simulink model "pv_simulink"  (R2025b)
settings: Solver=ode45  StartTime=0.0  StopTime=604900  RelTol=1e-3
InitFcn:
  | modellDatei   = get_param('pv_simulink', 'FileName');
  | projektWurzel = fileparts(fileparts(modellDatei));
  | addpath(projektWurzel);
  | 
  | p = init_parameters();
undefined symbols (not defined in the file): Tm_start
settings Model: Creator=T450s  LastModifiedBy=T450s

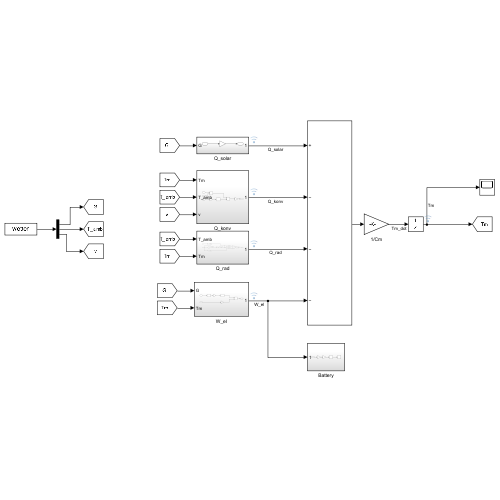
[thumbnail: Simulink's stored preview of the top-level diagram]
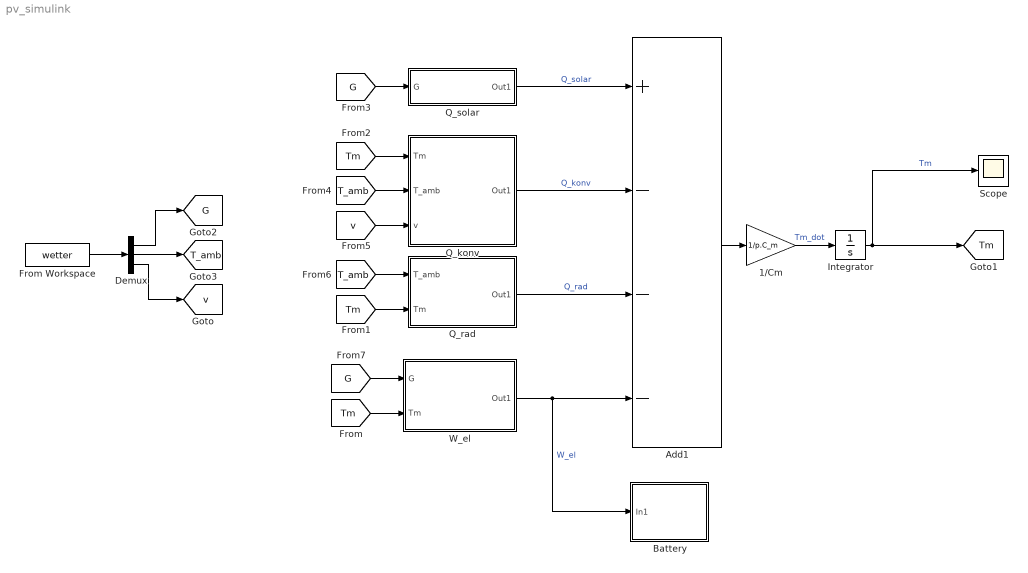
== system pv_simulink ==
  1/Cm : Gain  Gain=1/p.C_m
  Add1 : Sum  Inputs=+---
  Battery : Subsystem
  Demux : Demux  Outputs=3
  From Workspace : FromWorkspace  VariableName=wetter
  Integrator : Integrator  InitialCondition=Tm_start
  Q_konv : Subsystem
  Q_rad : Subsystem
  Q_solar : Subsystem
  Scope : Scope
      settings: ActiveDisplayYMinimum=-1  ActiveDisplayYMaximum=1
  W_el : Subsystem
  tag scope: G=global, T_amb=global, Tm=global, v=global
  wires:
  1/Cm/1 -> Integrator/1  "Tm_dot"
  Add1/1 -> 1/Cm/1
  Q_rad/1(Out1) -> Add1/3  "Q_rad"
  W_el/1(Out1) -> Battery/1(In1), Add1/4  "W_el"
  Q_konv/1(Out1) -> Add1/2  "Q_konv"
  Q_solar/1(Out1) -> Add1/1  "Q_solar"
  Integrator/1 -> Scope/1, [Tm]  "Tm"
  [Tm] -> W_el/2(Tm)
  [Tm] -> Q_rad/2(Tm)
  [Tm] -> Q_konv/1(Tm)
  [G] -> Q_solar/1(G)
  [T_amb] -> Q_konv/2(T_amb)
  [v] -> Q_konv/3(v)
  [T_amb] -> Q_rad/1(T_amb)
  [G] -> W_el/1(G)
  From Workspace/1 -> Demux/1
  Demux/1 -> [G]
  Demux/2 -> [T_amb]
  Demux/3 -> [v]

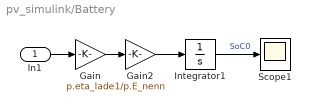
== system pv_simulink/Battery ==
  In1 : Inport
  Gain : Gain  Gain=p.eta_lade
  Gain2 : Gain  Gain=1/p.E_nenn
  Integrator1 : Integrator  InitialCondition=p.SoC0  LimitOutput=on  UpperSaturationLimit=1  LowerSaturationLimit=0
  Scope1 : Scope
      settings: ActiveDisplayYMinimum=0.10000000000000003  ActiveDisplayYMaximum=1.1
  wires:
  Gain2/1 -> Integrator1/1
  Gain/1 -> Gain2/1
  Integrator1/1 -> Scope1/1  "SoC0"
  In1/1 -> Gain/1

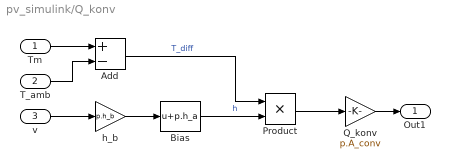
== system pv_simulink/Q_konv ==
  Tm : Inport
  T_amb : Inport  Port=2
  v : Inport  Port=3
  Add : Sum  Inputs=+-
  Bias : Bias  Bias=p.h_a  SaturateOnIntegerOverflow=off
  Product : Product
  Q_konv : Gain  Gain=p.A_conv
  h_b : Gain  Gain=p.h_b
  Out1 : Outport
  wires:
  T_amb/1 -> Add/2
  Add/1 -> Product/1  "T_diff"
  h_b/1 -> Bias/1
  Bias/1 -> Product/2  "h"
  Product/1 -> Q_konv/1
  Q_konv/1 -> Out1/1
  Tm/1 -> Add/1
  v/1 -> h_b/1

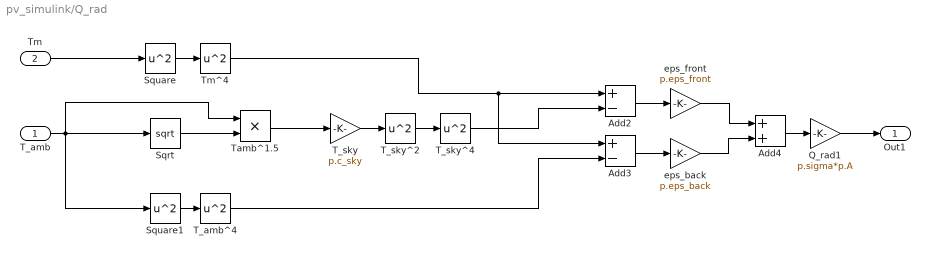
== system pv_simulink/Q_rad ==
  T_amb : Inport
  Tm : Inport  Port=2
  Add2 : Sum  Inputs=+-
  Add3 : Sum  Inputs=+-
  Add4 : Sum
  Q_rad1 : Gain  Gain=p.sigma*p.A
  Sqrt : Sqrt
  Square : Math  Operator=square
  Square1 : Math  Operator=square
  T_amb^4 : Math  Operator=square
  T_sky : Gain  Gain=p.c_sky
  T_sky^2 : Math  Operator=square
  T_sky^4 : Math  Operator=square
  Tamb^1.5 : Product
  Tm^4 : Math  Operator=square
  eps_back : Gain  Gain=p.eps_back
  eps_front : Gain  Gain=p.eps_front
  Out1 : Outport
  wires:
  eps_back/1 -> Add4/2
  T_amb^4/1 -> Add3/2
  Add3/1 -> eps_back/1
  Square1/1 -> T_amb^4/1
  Square/1 -> Tm^4/1
  Tamb^1.5/1 -> T_sky/1
  eps_front/1 -> Add4/1
  T_sky^4/1 -> Add2/2
  T_sky/1 -> T_sky^2/1
  Tm^4/1 -> Add3/1, Add2/1
  Add4/1 -> Q_rad1/1
  Sqrt/1 -> Tamb^1.5/2
  T_sky^2/1 -> T_sky^4/1
  Add2/1 -> eps_front/1
  T_amb/1 -> Tamb^1.5/1, Square1/1, Sqrt/1
  Q_rad1/1 -> Out1/1
  Tm/1 -> Square/1

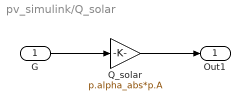
== system pv_simulink/Q_solar ==
  G : Inport
  Q_solar : Gain  Gain=p.alpha_abs*p.A
  Out1 : Outport
  wires:
  G/1 -> Q_solar/1
  Q_solar/1 -> Out1/1

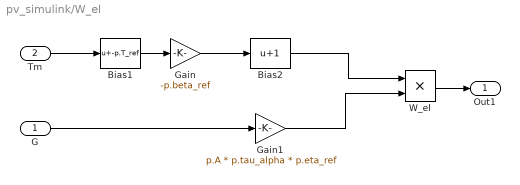
== system pv_simulink/W_el ==
  G : Inport
  Tm : Inport  Port=2
  Bias1 : Bias  Bias=-p.T_ref  SaturateOnIntegerOverflow=off
  Bias2 : Bias  Bias=1  SaturateOnIntegerOverflow=off
  Gain : Gain  Gain=-p.beta_ref
  Gain1 : Gain  Gain=p.A * p.tau_alpha * p.eta_ref
  W_el : Product
  Out1 : Outport
  wires:
  Gain/1 -> Bias2/1
  Tm/1 -> Bias1/1
  Gain1/1 -> W_el/2
  G/1 -> Gain1/1
  W_el/1 -> Out1/1
  Bias2/1 -> W_el/1
  Bias1/1 -> Gain/1
